simulink model "VCU_Software"  (R2024a)
settings: Solver=FixedStepDiscrete  StartTime=0  StopTime=2474  FixedStep=0.01  RelTol=2e-1  AbsTol=1e-1
libraries: autosarlibaprouting x20
settings Model: DataDictionary=VirtualVehicleTemplate.sldd  Creator=smuckati  LastModifiedBy=smuckati
settings SolverCC: AutoScaleAbsTol=off  SolverJacobianMethodControl=FullPerturbation  ZeroCrossAlgorithm=Adaptive  AlgebraicLoopSolver=TrustRegion  AutoInsertRateTranBlk=on  InsertRTBMode=Never (minimum delay)  DecoupledContinuousIntegration=on  MinimalZcImpactIntegration=on  MaxZcPerStep=1
settings OptimizationCC: DefaultParameterBehavior=Inlined  UseDivisionForNetSlopeComputation=on  GainParamInheritBuiltInType=on  UseFloatMulNetSlope=on  UseSpecifiedMinMax=on  InlineInvariantSignals=on  BitwiseOrLogicalOp=Bitwise operator  PassReuseOutputArgsAs=Individual arguments  ZeroExternalMemoryAtStartup=off  ZeroInternalMemoryAtStartup=off  NoFixptDivByZeroProtection=on  EfficientFloat2IntCast=on  LifeSpan=1  OptimizeBlockOrder=speed  DifferentSizesBufferReuse=on  EfficientTunableParamExpr=on
settings DebuggingCC: SignalInfNanChecking=error  ArtificialAlgebraicLoopMsg=none  MaskedZcDiagnostic=none  IgnoredZcDiagnostic=none  ParameterTunabilityLossMsg=error  UnconnectedInputMsg=warning  UnconnectedOutputMsg=warning  UnconnectedLineMsg=warning  PregeneratedLibrarySubsystemCodeDiagnostic=none  SubsystemReferenceDiagnosticForUnitTest=warning  ArithmeticOperatorsInVariantConditions=warning
settings HardwareCC: ProdBitPerPointer=32  ProdBitPerSizeT=32  ProdBitPerPtrDiffT=32  ProdLargestAtomicFloat=None  ProdWordSize=32  ProdHWDeviceType=Custom Processor->Custom Processor
settings ModelReferenceCC: UpdateModelReferenceTargets=IfOutOfDate  EnableRefExpFcnMdlSchedulingChecks=on  ModelReferenceMinAlgLoopOccurrences=on  PropagateSignalLabelsOutOfModel=off
settings SFSimCC: SimUseLocalCustomCode=off  SimGenImportedTypeDefs=on  MATLABDynamicMemAlloc=off  SimTargetLang=C++
settings RTWCC: Description=AUTOSAR Adaptive  SystemTargetFile=autosar_adaptive.tlc  GenCodeOnly=on  PackageGeneratedCodeAndArtifacts=on  TemplateMakefile=ert_default_tmf  GenerateReport=on  RTWUseLocalCustomCode=off  Toolchain=AUTOSAR Adaptive | CMake  BuildConfiguration=Faster Runs  IncludeHyperlinkInReport=on  DataTypeReplacement=CDataTypesFixedWidth  TargetLang=C++  GenerateTraceInfo=on  GenerateTraceReport=on  GenerateTraceReportSl=on  GenerateTraceReportSf=on  GenerateTraceReportEml=on  GenerateCodeMetricsReport=on  GenerateCodeReplacementReport=on  GPUComputeCapability=3.5  DLArmComputeVersion=19.05
settings CodeAppCC: ForceParamTrailComments=on  IgnoreCustomStorageClasses=off  MaxIdLength=63  OperatorAnnotations=on  SimulinkDataObjDesc=on  SFDataObjDesc=on  CustomSymbolStrGlobalVar=rt$N$M  CustomSymbolStrType=$N$M  CustomSymbolStrFcn=$N$M$F  CustomSymbolStrMacro=$N$M  InsertBlockDesc=on
settings AUTOSARAdaptiveTargetCC: TargetFcnLib=ansi_tfl_table_tmw.mat  GenFloatMathFcnCalls=NOT IN USE  TargetLangStandard=C++11 (ISO)  CodeReplacementLibrary=C++ Standard Library Mutex  UtilityFuncGeneration=Auto  MultiwordTypeDef=System defined  MultiwordLength=2048  DynamicStringBufferSize=256  GenerateFullHeader=on  InferredTypesCompatibility=off  GenerateSampleERTMain=off  GenerateTestInterfaces=off  ModelReferenceCompliant=on  ParMdlRefBuildCompliant=on  CompOptLevelCompliant=on  ConcurrentExecutionCompliant=on  IncludeMdlTerminateFcn=on  CombineOutputUpdateFcns=on  CombineSignalStateStructs=on  GroupInternalDataByFunction=off  SuppressErrorStatus=on  IncludeFileDelimiter=Auto  ERTCustomFileBanners=off  SupportAbsoluteTime=off  LogVarNameModifier=rt_  MatFileLogging=off  CodeInterfacePackaging=C++ class  PurelyIntegerCode=off  SupportNonFinite=off  SupportComplex=off  SupportContinuousTime=off  SupportNonInlinedSFcns=off  RemoveDisableFunc=off  RemoveResetFunc=on  SupportVariableSizeSignals=off  ParenthesesLevel=Nominal  CastingMode=Nominal  MATLABClassNameForMDSCustomization=Simulink.SoftwareTarget.TargetSpecificTriggerConfigurationBase  ModelStepFunctionPrototypeControlCompliant=off  CPPClassGenCompliant=on  AutosarCompliant=on  MDXCompliant=off  GRTInterface=off  GenerateAllocFcn=off  UseToolchainInfoCompliant=on  GenerateSharedConstants=on  CoderGroups=[]  AccessMethods=[]  LookupTableObjectStructAxisOrder=2,1,3,4,...  LUTObjectStructOrderExplicitValues=Size,Breakpoints,Table  LUTObjectStructOrderEvenSpacing=Size,Table,Breakpoints  ArrayLayout=Column-major  UnsupportedSFcnMsg=error  ERTHeaderFileRootName=$R$E  ERTSourceFileRootName=$R$E  ERTDataFileRootName=$R_data  InstructionSetFMA=off  OptimizeReductions=off  LogToMDFFile=off  GenerateASAP2=off  DSAsUniqueAccess=off  ExtMode=off  ExtModeTransport=0  ExtModeStaticAlloc=off  ExtModeAutomaticAllocSize=on  ExtModeMaxTrigDuration=10  ExtModeStaticAllocSize=1000000  ExtModeTesting=off  ExtModeMexFile=ext_comm  ExtModeIntrfLevel=Level1  InlinedParameterPlacement=NonHierarchical  TargetOS=BareBoardExample  MultiInstanceErrorCode=Error  RootIOFormat=Structure reference  RTWCAPISignals=off  RTWCAPIParams=off  RTWCAPIStates=off  RTWCAPIRootIO=off  ERTSrcFileBannerTemplate=ert_code_template.cgt  ERTHdrFileBannerTemplate=ert_code_template.cgt  ERTDataSrcFileTemplate=ert_code_template.cgt  ERTDataHdrFileTemplate=ert_code_template.cgt  ERTCustomFileTemplate=example_file_process.tlc  EnableDataOwnership=off  SignalDisplayLevel=10  ParamTuneLevel=10  GlobalDataDefinition=Auto  DataDefinitionFile=global.c  GlobalDataReference=Auto  ERTFilePackagingFormat=CompactWithDataFile  RateTransitionBlockCode=Inline  DataReferenceFile=global.h  PreserveExpressionOrder=off  PreserveIfCondition=off  ConvertIfToSwitch=on  PreserveExternInFcnDecls=on  PreserveStaticInFcnDecls=on  SuppressUnreachableDefaultCases=on  EnableSignedLeftShifts=on  EnableSignedRightShifts=on  ImplementImageWithCVMat=off  IndentStyle=K&R  IndentSize=2  NewlineStyle=Default  MaxLineWidth=80  EnableUserReplacementTypes=off  MaxIdInt64=INT64_MAX  MinIdInt64=INT64_MIN  MaxIdUint64=UINT64_MAX  MaxIdInt32=INT32_MAX  MinIdInt32=INT32_MIN  MaxIdUint32=UINT32_MAX  MaxIdInt16=INT16_MAX  MinIdInt16=INT16_MIN  MaxIdUint16=UINT16_MAX  MaxIdInt8=INT8_MAX  MinIdInt8=INT8_MIN  MaxIdUint8=UINT8_MAX  BooleanTrueId=true  BooleanFalseId=false  MemSecPackage=--- None ---  MemSecDataConstants=Default  MemSecDataIO=Default  MemSecDataInternal=Default  MemSecDataParameters=Default  MemSecFuncInitTerm=Default  MemSecFuncExecute=Default  MemSecFuncSharedUtil=Default  GroupConstants=Default  GroupRootInputs=Default  GroupRootOutputs=Default  GroupInternal=Default  GroupParameters=Default  GroupDataTransfer=Default  GroupSharedLocalDataStores=Default  GroupInstanceSpecificParameters=Default  GroupModelData=Default  ArrayContainerType=std::array  AutosarSchemaVersion=R20-11  AutosarMaxShortNameLength=128  AdaptiveAutosarXCPServerTransportLayer=None  AdaptiveAutosarXCPServerTCPIPAddress=127.0.0.1  AdaptiveAutosarXCPServerPort=17725  AdaptiveAutosarXCPServerVerbosity=off  AdaptiveAutosarUseCustomXCPServer=off

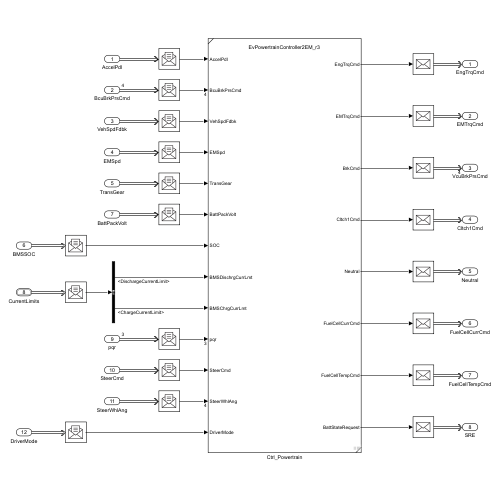
[thumbnail: Simulink's stored preview of the top-level diagram]
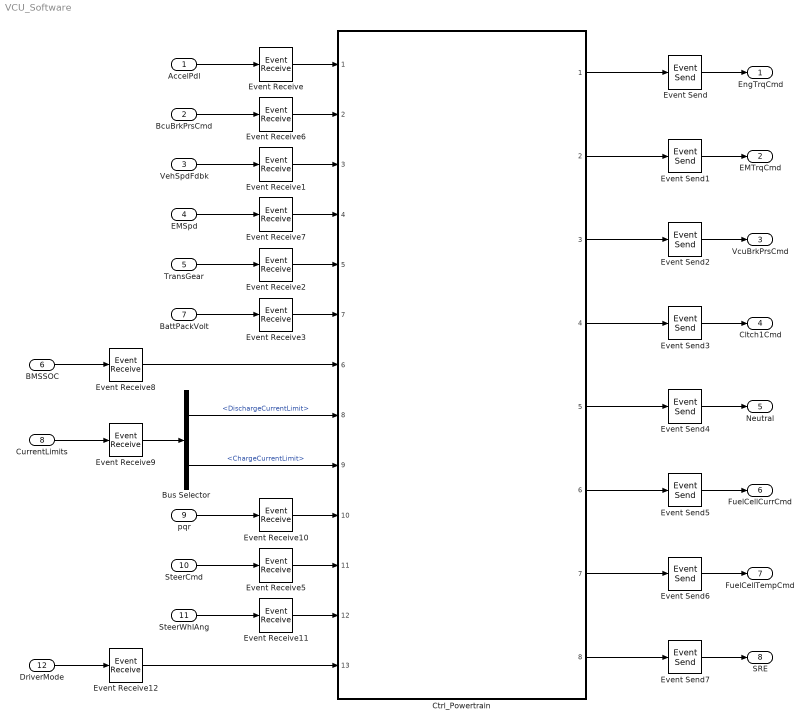
== system VCU_Software ==
  AccelPdl : Inport  OutputPortMessageModes=m  OutDataTypeStr=double  PortDimensions=1
  BcuBrkPrsCmd : Inport  OutputPortMessageModes=m  Port=2  OutDataTypeStr=double  PortDimensions=4
  VehSpdFdbk : Inport  OutputPortMessageModes=m  Port=3  OutDataTypeStr=double  PortDimensions=1
  EMSpd : Inport  OutputPortMessageModes=m  Port=4  OutDataTypeStr=double
  TransGear : Inport  OutputPortMessageModes=m  Port=5  OutDataTypeStr=double  PortDimensions=1
  BMSSOC : Inport  OutputPortMessageModes=m  Port=6
  BattPackVolt : Inport  OutputPortMessageModes=m  Port=7
  CurrentLimits : Inport  OutputPortMessageModes=m  Port=8  OutDataTypeStr=Bus: BattCurLims  BusOutputAsStruct=on
  pqr : Inport  OutputPortMessageModes=m  Port=9  PortDimensions=3
  SteerCmd : Inport  OutputPortMessageModes=m  Port=10
  SteerWhlAng : Inport  OutputPortMessageModes=m  Port=11
  DriverMode : Inport  OutputPortMessageModes=m  Port=12  OutDataTypeStr=Enum: DriverMode
  Bus Selector : BusSelector  OutputSignals=DischargeCurrentLimit,ChargeCurrentLimit
  Ctrl_Powertrain : Subsystem  ReferencedSubsystem=EvPowertrainController2EM_r3
      settings: PortSchema="{\"entries\":[{\"content\":{\"sides\":[{\"content\":{\"connectorIds\":[\"In1\",\"In2\",\"In3\",\"In4\",\"In5\",\"In7\",\"In6\",\"In8\",\"In9\",\"In10\",\"In11\",\"In12\",\"In13\"]},\"type\":\"ConnectorPlacement.EquallySpacedRectSide\",\"uuid\":\"d88b7e8a-a6be-4aa9-9ace-8036a966e6f2\"},{\"content\":{\"connectorIds\":[\"Out1\",\"Out2\",\"Out3\",\"Out4\",\"Out5\",\"Out6\",\"Out7\",\"Out8\"],\"side\":\"RIGHT\"},\"type\":\"ConnectorPlacement.EquallySpacedRectSide\",\"uuid\":\"7a9afc9b-f53d-4f8b-a416-aba0864c8b66\"},{\"content\":{\"side\":\"TOP\"},\"type\":\"ConnectorPlacement.EquallySpacedRectSide\",\"uuid\":\"8ca5d5ff-bf9d-4962-9c01-4f7cca42c215\"}]},\"type\":\"ConnectorPlacement.EquallySpacedConnector\",\"uuid\":\"3368383a-4578-43b5-996f-32614659e186\"}],\"packageUris\":[\"http://schema.mathworks.com/mf0/Connector/R2020b\"],\"version\":\"1.0\"}"
  Event Receive{,1..3,5..12} (12 alike) : autosarlibaprouting/Event Receive
  Event Send{,1..7} (8 alike) : autosarlibaprouting/Event Send
  EngTrqCmd : Outport  InputPortMessageModes=m  OutDataTypeStr=double  PortDimensions=1  VectorParamsAs1DForOutWhenUnconnected=off
  EMTrqCmd : Outport  InputPortMessageModes=m  Port=2  OutDataTypeStr=double  VectorParamsAs1DForOutWhenUnconnected=off
  VcuBrkPrsCmd : Outport  InputPortMessageModes=m  Port=3  OutDataTypeStr=double  PortDimensions=4  VectorParamsAs1DForOutWhenUnconnected=off
  Cltch1Cmd : Outport  InputPortMessageModes=m  Port=4  OutDataTypeStr=double  PortDimensions=1  VectorParamsAs1DForOutWhenUnconnected=off
  Neutral : Outport  InputPortMessageModes=m  Port=5  OutDataTypeStr=double  PortDimensions=1  VectorParamsAs1DForOutWhenUnconnected=off
  FuelCellCurrCmd : Outport  InputPortMessageModes=m  Port=6  OutDataTypeStr=double  PortDimensions=1
  FuelCellTempCmd : Outport  InputPortMessageModes=m  Port=7  OutDataTypeStr=double  PortDimensions=1
  SRE : Outport  InputPortMessageModes=m  Port=8  OutDataTypeStr=Enum: SRE  PortDimensions=1
  wires:
  AccelPdl/1 -> Event Receive/1
  BMSSOC/1 -> Event Receive8/1
  Event Send2/1 -> VcuBrkPrsCmd/1
  pqr/1 -> Event Receive10/1
  VehSpdFdbk/1 -> Event Receive1/1
  BcuBrkPrsCmd/1 -> Event Receive6/1
  SteerCmd/1 -> Event Receive5/1
  EMSpd/1 -> Event Receive7/1
  Event Receive5/1 -> Ctrl_Powertrain/11
  Event Receive6/1 -> Ctrl_Powertrain/2
  TransGear/1 -> Event Receive2/1
  BattPackVolt/1 -> Event Receive3/1
  SteerWhlAng/1 -> Event Receive11/1
  DriverMode/1 -> Event Receive12/1
  Event Send/1 -> EngTrqCmd/1
  Event Receive9/1 -> Bus Selector/1
  Event Receive/1 -> Ctrl_Powertrain/1
  Event Send1/1 -> EMTrqCmd/1
  Event Receive1/1 -> Ctrl_Powertrain/3
  Event Receive7/1 -> Ctrl_Powertrain/4
  Event Receive12/1 -> Ctrl_Powertrain/13
  Event Receive2/1 -> Ctrl_Powertrain/5
  Event Receive3/1 -> Ctrl_Powertrain/7
  Bus Selector/2 -> Ctrl_Powertrain/9  "<ChargeCurrentLimit>"
  Event Receive10/1 -> Ctrl_Powertrain/10
  Event Receive11/1 -> Ctrl_Powertrain/12
  Ctrl_Powertrain/3 -> Event Send2/1
  Ctrl_Powertrain/4 -> Event Send3/1
  Ctrl_Powertrain/5 -> Event Send4/1
  Ctrl_Powertrain/6 -> Event Send5/1
  Ctrl_Powertrain/7 -> Event Send6/1
  Ctrl_Powertrain/8 -> Event Send7/1
  Event Send4/1 -> Neutral/1
  Event Send3/1 -> Cltch1Cmd/1
  Event Send5/1 -> FuelCellCurrCmd/1
  Event Send6/1 -> FuelCellTempCmd/1
  Event Send7/1 -> SRE/1
  CurrentLimits/1 -> Event Receive9/1
  Bus Selector/1 -> Ctrl_Powertrain/8  "<DischargeCurrentLimit>"
  Ctrl_Powertrain/1 -> Event Send/1
  Ctrl_Powertrain/2 -> Event Send1/1
  Event Receive8/1 -> Ctrl_Powertrain/6
